simulink model "s_3d_crane_tower_pos_cntrl"  (Simulink 6.6)
settings: Solver=FixedStepDiscrete  StartTime=0.0  StopTime=10  FixedStep=0.001  RelTol=1e-3
values from neighbouring files (symbols this model uses):
  A_T = A    [setup_3d_crane.m]
  B_T = B    [setup_3d_crane.m]
  C_T = C    [setup_3d_crane.m]
  D_T = D    [setup_3d_crane.m]
  IMAX_AMP = 7    [setup_3d_crane.m]
  K_T = lqr(A_T,B_T,Q_T,R_T)    [setup_3d_crane.m]
  wf_gamma = 2 * pi * 2.0    (= 12.5663706144)    [setup_3d_crane.m]
  wf_theta = 2 * pi * 50    (= 314.159265359)    [setup_3d_crane.m]
undefined symbols (not defined in the file or in its folder): qc_get_step_size
libraries: simulink_extras x4, quarc_library x4, simulink x2
settings Model: Creator=MLevis  LastModifiedBy=MLevis  ExtModeTrigDuration=10000
settings SolverCC: PositivePriorityOrder=on
settings RTWCC: SystemTargetFile=quarc_windows.tlc  TemplateMakefile=quarc_default_tmf  Description=QuaRC Win32 Target  ProcessScript=quarc_windows_make_rtw_hook
settings STFCustomTargetCC: TargetFcnLib=ansi_tfl_tmw.mat  TargetPreCompLibLocation=C:\DOCUME~1\ALLUSE~1\APPLIC~1\QuaRC\lib\2007a\windows\release  GenFloatMathFcnCalls=ANSI_C  SystemTargetFile=quarc_windows.tlc
settings GRTTargetCC: TargetPreCompLibLocation=C:\DOCUME~1\ALLUSE~1\APPLIC~1\QuaRC\lib\2007a\windows\release  MatFileLogging=off  ExtMode=on  ExtModeMexFile=quarc_comm

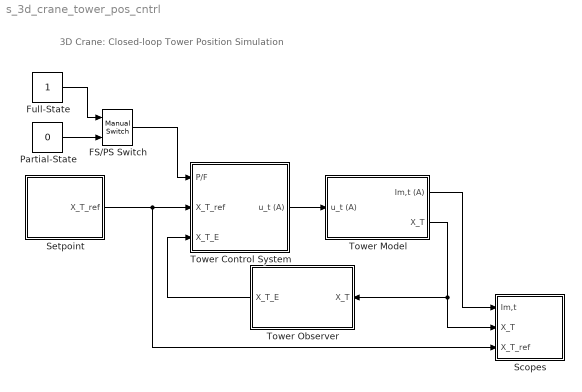
== system s_3d_crane_tower_pos_cntrl ==
  note: 3D Crane: Closed-loop Tower Position Simulation
  FS/PS Switch : simulink/Signal Routing/Manual Switch  SystemSampleTime=-1  sw=1  action=0  varsize=off
  Full-State : Constant
  Partial-State : Constant  Value=0
  Scopes : Subsystem
  Setpoint : Subsystem
  Tower Control System : Subsystem
  Tower Model : Subsystem
  Tower Observer : Subsystem  Orientation=left
  wires:
  Setpoint/1(X_T_ref) -> Scopes/3(X_T_ref), Tower Control System/2(X_T_ref)
  Tower Control System/1(u_t (A)) -> Tower Model/1(u_t (A))
  Full-State/1 -> FS/PS Switch/1
  Partial-State/1 -> FS/PS Switch/2
  FS/PS Switch/1 -> Tower Control System/1(P/F)
  Tower Model/2(X_T) -> Tower Observer/1(X_T), Scopes/2(X_T)
  Tower Model/1(Im,t (A)) -> Scopes/1(Im,t)
  Tower Observer/1(X_T_E) -> Tower Control System/3(X_T_E)

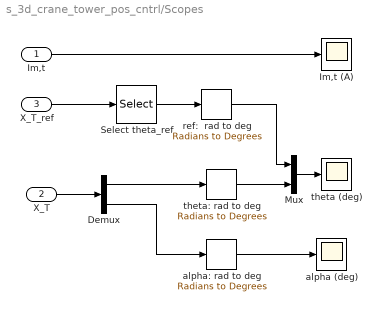
== system s_3d_crane_tower_pos_cntrl/Scopes ==
  Im,t : Inport
  X_T : Inport  Port=2
  X_T_ref : Inport  Port=3
  Demux : Demux  Outputs=2
  Im,t (A) : Scope
      settings: TimeRange=10  YMin=-0.4  YMax=1  SaveName=ScopeData4
  Mux : Mux  Inputs=2
  Select theta_ref : Selector  IndexOptions=Index vector (dialog)  Indices=1  OutputSizes=1  InputPortWidth=4
  alpha (deg) : Scope
      settings: TimeRange=10  YMin=-6  YMax=8
  alpha: rad to deg : simulink_extras/Transformations/Radians to Degrees  SystemSampleTime=-1
  ref:  rad to deg : simulink_extras/Transformations/Radians to Degrees  SystemSampleTime=-1
  theta (deg) : Scope
      settings: TimeRange=10  YMin=0  YMax=70
  theta: rad to deg : simulink_extras/Transformations/Radians to Degrees  SystemSampleTime=-1
  wires:
  Select theta_ref/1 -> ref:  rad to deg/1
  Im,t/1 -> Im,t (A)/1
  X_T/1 -> Demux/1
  X_T_ref/1 -> Select theta_ref/1
  Demux/2 -> alpha: rad to deg/1
  Demux/1 -> theta: rad to deg/1
  alpha: rad to deg/1 -> alpha (deg)/1
  theta: rad to deg/1 -> Mux/2
  ref:  rad to deg/1 -> Mux/1
  Mux/1 -> theta (deg)/1

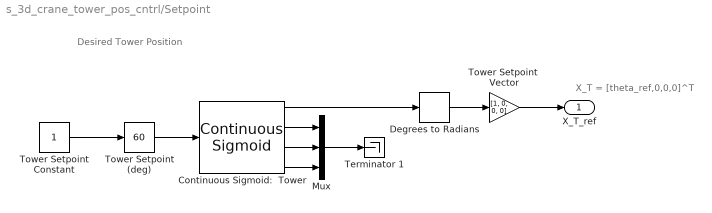
== system s_3d_crane_tower_pos_cntrl/Setpoint ==
  note: X_T = [theta_ref,0,0,0]^T
  note: Desired Tower Position
  Continuous Sigmoid:  Tower : quarc_library/Sources/Sigmoids/Continuous Sigmoid  params_source=Internal (dialog parameters)  max_velocity=75  max_acceleration=45  initial_position=0  initial_velocity=0  hold_off=0.5  input_sample_time=-1  output_sample_time=qc_get_step_size
  Degrees to Radians : simulink_extras/Transformations/Degrees to Radians  SystemSampleTime=-1
  Mux : Mux  Inputs=3
  Terminator 1 : Terminator
  Tower Setpoint (deg) : simulink/Math Operations/Slider Gain  SystemSampleTime=-1  low=-120  gain=60  high=120
  "Tower Setpoint Constant " : Constant
  Tower Setpoint  Vector : Gain  Gain=[1, 0, 0, 0]
  X_T_ref : Outport
  wires:
  Continuous Sigmoid:  Tower/1 -> Degrees to Radians/1
  "Tower Setpoint Constant "/1 -> Tower Setpoint (deg)/1
  Tower Setpoint (deg)/1 -> Continuous Sigmoid:  Tower/1
  Degrees to Radians/1 -> Tower Setpoint  Vector/1
  Continuous Sigmoid:  Tower/2 -> Mux/1
  Continuous Sigmoid:  Tower/3 -> Mux/2
  Continuous Sigmoid:  Tower/4 -> Mux/3
  Mux/1 -> Terminator 1/1
  Tower Setpoint  Vector/1 -> X_T_ref/1

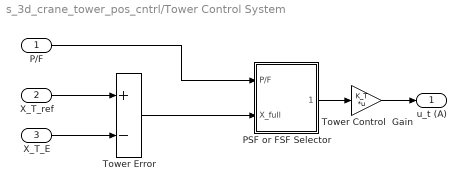
== system s_3d_crane_tower_pos_cntrl/Tower Control System ==
  P/F : Inport
  X_T_ref : Inport  Port=2
  X_T_E : Inport  Port=3
  PSF or FSF Selector : Subsystem
  Tower Control  Gain : Gain  Gain=K_T  Multiplication=Matrix(K*u)
  Tower Error : Sum  Inputs=+-  OutScaling=2^-10
  u_t (A) : Outport
  wires:
  Tower Control  Gain/1 -> u_t (A)/1
  X_T_ref/1 -> Tower Error/1
  X_T_E/1 -> Tower Error/2
  P/F/1 -> PSF or FSF Selector/1(P/F)
  Tower Error/1 -> PSF or FSF Selector/2(X_full)
  PSF or FSF Selector/1(X_out) -> Tower Control  Gain/1

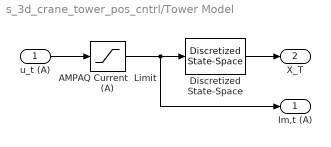
== system s_3d_crane_tower_pos_cntrl/Tower Model ==
  u_t (A) : Inport
  AMPAQ Current  Limit (A) : Saturate  UpperLimit=IMAX_AMP  LowerLimit=-IMAX_AMP  SampleTime=qc_get_step_size
  Discretized State-Space : quarc_library/Discrete/Discretized State-Space  SystemSampleTime=-1  A=A_T  B=B_T  C=C_T  D=D_T  x0=[0]  method=tustin  Ts=qc_get_step_size
  Im,t (A) : Outport
  X_T : Outport  Port=2
  wires:
  Discretized State-Space/1 -> X_T/1
  AMPAQ Current  Limit (A)/1 -> Im,t (A)/1, Discretized State-Space/1
  u_t (A)/1 -> AMPAQ Current  Limit (A)/1

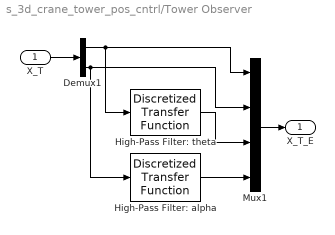
== system s_3d_crane_tower_pos_cntrl/Tower Observer ==
  X_T : Inport
  Demux1 : Demux  Outputs=2
  High-Pass Filter: alpha : quarc_library/Discrete/Discretized Transfer Function  SystemSampleTime=-1  num=[wf_gamma 0]  den=[1 wf_gamma]  method=tustin  Ts=qc_get_step_size
  High-Pass Filter: theta : quarc_library/Discrete/Discretized Transfer Function  SystemSampleTime=-1  num=[wf_theta 0]  den=[1 wf_theta]  method=tustin  Ts=qc_get_step_size
  Mux1 : Mux
  X_T_E : Outport
  wires:
  Demux1/1 -> Mux1/1, High-Pass Filter: theta/1
  Demux1/2 -> Mux1/2, High-Pass Filter: alpha/1
  High-Pass Filter: theta/1 -> Mux1/3
  High-Pass Filter: alpha/1 -> Mux1/4
  X_T/1 -> Demux1/1
  Mux1/1 -> X_T_E/1

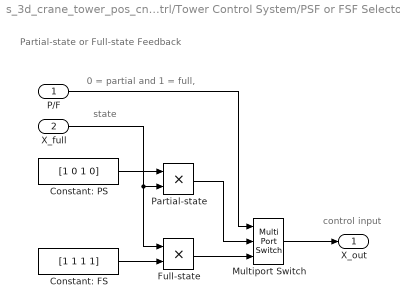
== system s_3d_crane_tower_pos_cntrl/Tower Control System/PSF or FSF Selector ==
  note: control input
  note: state
  note: 0 = partial and 1 = full,
  note: Partial-state or Full-state Feedback
  P/F : Inport
  X_full : Inport  Port=2
  Constant: FS : Constant  Value=[1 1 1 1]
  Constant: PS : Constant  Value=[1 0 1 0]
  Full-state : Product  RndMeth=Zero
  Multiport Switch : MultiPortSwitch  Inputs=2  zeroidx=on
  Partial-state : Product  RndMeth=Zero
  X_out : Outport
  wires:
  X_full/1 -> Full-state/1, Partial-state/2
  P/F/1 -> Multiport Switch/1
  Multiport Switch/1 -> X_out/1
  Full-state/1 -> Multiport Switch/3
  Partial-state/1 -> Multiport Switch/2
  Constant: PS/1 -> Partial-state/1
  Constant: FS/1 -> Full-state/2
